simulink model "sim_SS_H2DF_2024a_GRU"  (R2024a)
settings: Solver=FixedStepAuto  StartTime=0.0  StopTime=4899  FixedStep=1  RelTol=1e-3  EnableMultiTasking=on
model workspace (MAT data in the model file):
  enable_IMEP_noise = 100
  enable_IMEP_offset = 1
values from neighbouring files (symbols this model uses):
  C2C_NMPC = init_C2C_NMPC_H2DF(C2C_NMPC.expdata)    [run_SS_H2DF_control.m]
undefined symbols (not defined in the file or in its folder): cost_length, horizon_length, y_ref_buf
libraries: matrix_library x3
(part 3 of 3)

== matlab function sim_SS_H2DF_2024a_GRU/dynamics/C2C_NMPC/C2C_NMPC_n3/constraints (no soft)/MATLAB Function2 ==
  data: value input; vector output; length input; init_vector input
function vector = fcn(value, length, init_vector)
init_vector(1:(size(value,1)*length)) = repmat(value, length, 1);
vector = init_vector;

== matlab function sim_SS_H2DF_2024a_GRU/dynamics/C2C_NMPC/C2C_NMPC_n3/constraints (no soft)/MATLAB Function3 ==
  data: value input; vector output; length input; init_vector input
function vector = fcn(value, length, init_vector)
init_vector(1:(size(value,1)*length)) = repmat(value, length, 1);
vector = init_vector;

== matlab function sim_SS_H2DF_2024a_GRU/dynamics/C2C_NMPC/C2C_NMPC_n3/constraints (no soft)/MATLAB Function4 ==
  data: value input; vector output; length input; init_vector input
function vector = fcn(value, length, init_vector)
init_vector(1:(size(value,1)*length)) = repmat(value, length, 1);
vector = init_vector;

== matlab function sim_SS_H2DF_2024a_GRU/dynamics/C2C_NMPC/C2C_NMPC_n3/constraints (no soft)/MATLAB Function5 ==
  data: value input; vector output; length input; init_vector input
function vector = fcn(value, length, init_vector)
init_vector(1:(size(value,1)*length)) = repmat(value, length, 1);
vector = init_vector;
